simulink model "n2grad"  (R2015b)
settings: Solver=VariableStepAuto  StartTime=0.0  StopTime=10.0  RelTol=1e-3
settings Model: Creator=Joern  LastModifiedBy=Joern

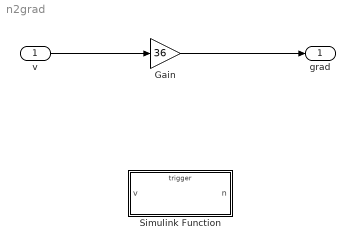
== system n2grad ==
  v : Inport
  Gain : Gain  Gain=36
  Simulink Function : Subsystem  TreatAsAtomicUnit=on
  grad : Outport
  wires:
  v/1 -> Gain/1
  Gain/1 -> grad/1

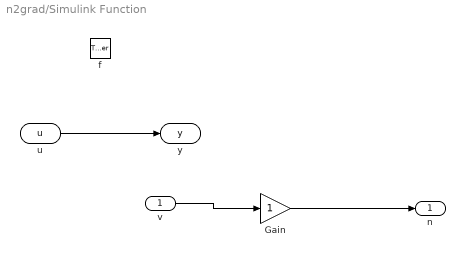
== system n2grad/Simulink Function ==
  v : Inport
  f : TriggerPort  TriggerType=function-call  IsSimulinkFunction=on  FunctionName=f
  Gain : Gain
  u : ArgIn  DisableCoverage=on  ArgumentName=u
  y : ArgOut  DisableCoverage=on  ArgumentName=y
  n : Outport
  wires:
  u/1 -> y/1
  v/1 -> Gain/1
  Gain/1 -> n/1
